simulink model "Identversuch_stabil"  (Simulink 7.0)
settings: Solver=ode45  StartTime=0.0  StopTime=tend  FixedStep=0.001  RelTol=1e-3
values from neighbouring files (symbols this model uses):
  t_prbs = 0.1    [SPI2_Uebung2_SimonsLoesung.m]
  Ts = 0.005    [SPI2_Uebung2_SimonsLoesung.m]    (also in testHannWindow.m = 0.1)
libraries: simulink_extras x2, simulink x1
settings Model: Creator=dominik  LastModifiedBy=dominik

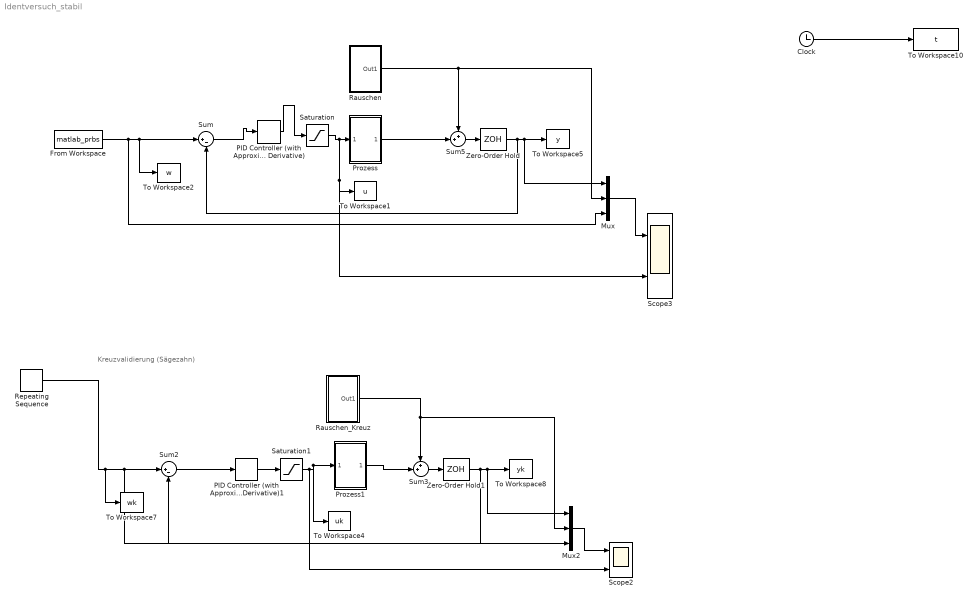
== system Identversuch_stabil ==
  note: Kreuzvalidierung (Sägezahn)
  Clock : Clock
      settings: Decimation=10
  From Workspace : FromWorkspace  VariableName=matlab_prbs  SampleTime=t_prbs  Interpolate=off  OutputAfterFinalValue=Setting to zero
  Mux : Mux  Inputs=3
  Mux2 : Mux  Inputs=3
  PID Controller (with Approximate Derivative) : simulink_extras/Additional Linear/PID Controller (with Approximate Derivative)  SystemSampleTime=-1  P=0.05  I=0.05  D=1  N=0.1
  PID Controller (with Approximate Derivative)1 : simulink_extras/Additional Linear/PID Controller (with Approximate Derivative)  SystemSampleTime=-1  P=0.05  I=0.05  D=1  N=0.1
  Prozess : Subsystem
  Prozess1 : Subsystem
  Rauschen : Subsystem
  Rauschen_Kreuz : Subsystem
  Repeating Sequence : simulink/Sources/Repeating Sequence  SystemSampleTime=-1  rep_seq_t=[0 2]  rep_seq_y=[0 0.1]
  Saturation : Saturate  UpperLimit=1  LowerLimit=-1  OutDataType=sfix(16)  OutScaling=2^0
  Saturation1 : Saturate  UpperLimit=1  LowerLimit=-1  OutDataType=sfix(16)  OutScaling=2^0
  Scope2 : Scope  NumInputPorts=2
      settings: TimeRange=10  YMin=-2~-0.01  YMax=1.25~0.01  SaveName=ScopeData2
  Scope3 : Scope  NumInputPorts=2
      settings: TimeRange=10  YMin=-2~-0.01  YMax=1.25~0.01
  Sum : Sum  Inputs=|+-  OutDataType=sfix(16)  OutScaling=2^0
  Sum2 : Sum  Inputs=|+-  OutDataType=sfix(16)  OutScaling=2^0
  Sum3 : Sum  Inputs=++|  OutDataType=sfix(16)  OutScaling=2^0
  Sum5 : Sum  Inputs=++|  OutDataType=sfix(16)  OutScaling=2^0
  To Workspace1 : ToWorkspace  VariableName=u  SampleTime=Ts  SaveFormat=Array
  To Workspace10 : ToWorkspace  VariableName=t  SampleTime=Ts  SaveFormat=Array
  To Workspace2 : ToWorkspace  VariableName=w  SampleTime=Ts  SaveFormat=Array
  To Workspace4 : ToWorkspace  VariableName=uk  SampleTime=Ts  SaveFormat=Array
  To Workspace5 : ToWorkspace  VariableName=y  SampleTime=Ts  SaveFormat=Array
  To Workspace7 : ToWorkspace  VariableName=wk  SampleTime=Ts  SaveFormat=Array
  To Workspace8 : ToWorkspace  VariableName=yk  SampleTime=Ts  SaveFormat=Array
  Zero-Order Hold : ZeroOrderHold  SampleTime=Ts
  Zero-Order Hold1 : ZeroOrderHold  SampleTime=Ts
  wires:
  From Workspace/1 -> Sum/1, Mux/3, To Workspace2/1
  Sum/1 -> PID Controller (with Approximate Derivative)/1
  Prozess/1(Out1) -> Sum5/2
  Clock/1 -> To Workspace10/1
  Sum5/1 -> Zero-Order Hold/1
  Mux/1 -> Scope3/1
  Rauschen/1(Out1) -> Sum5/1, Mux/2
  Zero-Order Hold/1 -> Mux/1, To Workspace5/1, Sum/2
  Sum2/1 -> PID Controller (with Approximate Derivative)1/1
  Sum3/1 -> Zero-Order Hold1/1
  Mux2/1 -> Scope2/1
  Rauschen_Kreuz/1(Out1) -> Sum3/1, Mux2/2
  Zero-Order Hold1/1 -> Mux2/1, To Workspace8/1, Sum2/2
  PID Controller (with Approximate Derivative)/1 -> Saturation/1
  Saturation/1 -> To Workspace1/1, Scope3/2, Prozess/1(In1)
  Repeating Sequence/1 -> To Workspace7/1, Sum2/1, Mux2/3
  PID Controller (with Approximate Derivative)1/1 -> Saturation1/1
  Saturation1/1 -> Prozess1/1(In1), To Workspace4/1, Scope2/2
  Prozess1/1(Out1) -> Sum3/2

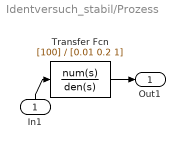
== system Identversuch_stabil/Prozess ==
  In1 : Inport  Orientation=up
  Transfer Fcn : TransferFcn  Description=System  Numerator=[100]  Denominator=[0.01 0.2 1]
  Out1 : Outport
  wires:
  In1/1 -> Transfer Fcn/1
  Transfer Fcn/1 -> Out1/1

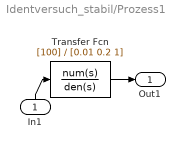
== system Identversuch_stabil/Prozess1 ==
  In1 : Inport  Orientation=up
  Transfer Fcn : TransferFcn  Description=System  Numerator=[100]  Denominator=[0.01 0.2 1]
  Out1 : Outport
  wires:
  In1/1 -> Transfer Fcn/1
  Transfer Fcn/1 -> Out1/1

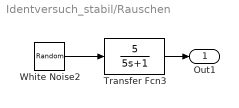
== system Identversuch_stabil/Rauschen ==
  Transfer Fcn3 : TransferFcn  Numerator=5  Denominator=[5 1]
  White Noise2 : RandomNumber  Variance=0.7^2  Seed=[2316]  SampleTime=0
  Out1 : Outport
  wires:
  White Noise2/1 -> Transfer Fcn3/1
  Transfer Fcn3/1 -> Out1/1

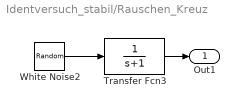
== system Identversuch_stabil/Rauschen_Kreuz ==
  Transfer Fcn3 : TransferFcn  Denominator=[1 1]
  White Noise2 : RandomNumber  Variance=0.7^2  Seed=[121201]  SampleTime=0
  Out1 : Outport
  wires:
  White Noise2/1 -> Transfer Fcn3/1
  Transfer Fcn3/1 -> Out1/1
